simulink model "APPS_Br_Plaus"  (R2021a)
settings: Solver=VariableStepAuto  StartTime=0.0  StopTime=10.0  RelTol=1e-3
settings Model: Creator=shind  LastModifiedBy=shind

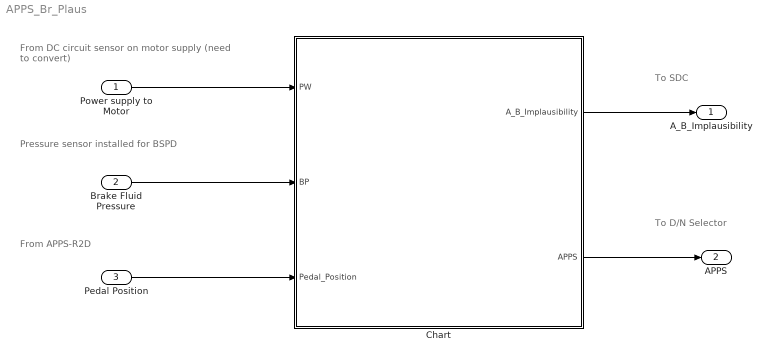
== system APPS_Br_Plaus ==
  note: To SDC
  note: Pressure sensor installed for
      | BSPD
  note: From DC circuit sensor on motor
      | supply (need to convert)
  note: From APPS-R2D
  note: To D/N Selector
  Power supply to Motor : Inport
  Brake Fluid Pressure : Inport  Port=2
  Pedal Position : Inport  Port=3
  Chart : Stateflow chart  TreatAsAtomicUnit=on
  A_B_Implausibility : Outport
  APPS : Outport  Port=2
  wires:
  Power supply to Motor/1 -> Chart/1(PW)
  Brake Fluid Pressure/1 -> Chart/2(BP)
  Pedal Position/1 -> Chart/3(Pedal_Position)
  Chart/1(A_B_Implausibility) -> A_B_Implausibility/1
  Chart/2(APPS) -> APPS/1

== stateflow chart APPS_Br_Plaus/Chart ==
  state Normal
    entry:
    A_B_Implausibility=0;
    APPS=Pedal_Position;
  state APPS_Brake_Implausible
    entry:
    A_B_Implausibility=1;
    APPS=0;
  state Time_Check
  (default) -> Normal
  Normal -> Time_Check : [BP>=30 && PW>=5000]
  Time_Check -> APPS_Brake_Implausible [order 1] : after(500,msec)
  Time_Check -> Normal [order 2] : [BP<30 || PW<5000]
  APPS_Brake_Implausible -> Normal : [Pedal_Position==0]
  data: A_B_Implausibility output; PW input; BP input; Pedal_Position input; APPS output
